simulink model "StateSpace"  (R2018b)
settings: Solver=VariableStepAuto  StartTime=0.0  StopTime=10.0  RelTol=1e-3
values from neighbouring files (symbols this model uses):
  A = [-7.6258  0; 1  0]    [stateSpaceData.mat]
  B = [1 0]    [stateSpaceData.mat]
  C = [0 162.7435]    [stateSpaceData.mat]
  D = 0    [stateSpaceData.mat]
  K = [-1.6258 11]    [stateSpaceData.mat]    (also in toStateSpace.m = [Kx(1) Kx(2)]; toStateSpaceAntiWindup.m = [Kx(1) Kx(2)])
  L = [80.8124614847 1.48930187688]    [stateSpaceData.mat]    (also in toStateSpace.m = acker(A', C', [polo1, polo2])'; toStateSpaceAntiWindup.m = acker(A', C', [polo1, polo2])')
settings Model: Creator=lucas  LastModifiedBy=lucas

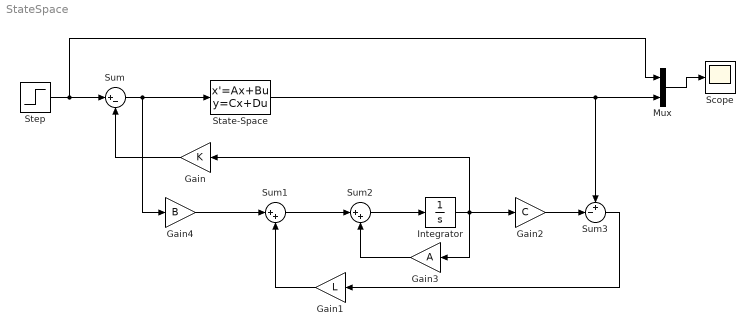
== system StateSpace ==
  Gain : Gain  Gain=K
  Gain1 : Gain  Gain=L
  Gain2 : Gain  Gain=C
  Gain3 : Gain  Gain=A
  Gain4 : Gain  Gain=B
  Integrator : Integrator
  Mux : Mux  Inputs=2
  Scope : Scope
  State-Space : StateSpace  A=A  B=B  C=C  D=D  InitialCondition=0
  Step : Step  After=20  SampleTime=0
  Sum : Sum  Inputs=|+-
  Sum1 : Sum  Inputs=|++
  Sum2 : Sum  Inputs=|++
  Sum3 : Sum  Inputs=+-|
  wires:
  Mux/1 -> Scope/1
  Step/1 -> Mux/1, Sum/1
  State-Space/1 -> Sum3/1, Mux/2
  Sum/1 -> Gain4/1, State-Space/1
  Gain/1 -> Sum/2
  Integrator/1 -> Gain3/1, Gain2/1, Gain/1
  Gain2/1 -> Sum3/2
  Gain3/1 -> Sum2/2
  Sum2/1 -> Integrator/1
  Sum3/1 -> Gain1/1
  Gain1/1 -> Sum1/2
  Sum1/1 -> Sum2/1
  Gain4/1 -> Sum1/1
